simulink model "Simulation_full_Matlab"  (R2024b)
settings: Solver=ode23tb  StartTime=0.0  StopTime=10  MaxStep=1e-5  RelTol=1e-4
InitFcn:
  | Motor_data_IM_R;
undefined symbols (not defined in the file): DiscIntNeverNeededParam, f_n, imr_min, J, j, K_r, K_s, ki, Ki_flux, Ki_w, kp, Kp_flux, Kp_w, L_sigma_r, L_sigma_s, lim, p, P_IN_VA, P_m_n, R_r, R_s, Tau_r, Ts, V_dc, V_ll_n, w_n, wr_n
libraries: slpidlib x2, spsCurrentMeasurementLib x2, spsAsynchronousMachineSIUnitsLib x1, spsDCVoltageSourceLib x1, simulink x1, spsSeriesRLCBranchLib x1, spsUniversalBridgeLib x1, sps_lib x1
settings Model: Creator=dario  LastModifiedBy=dario

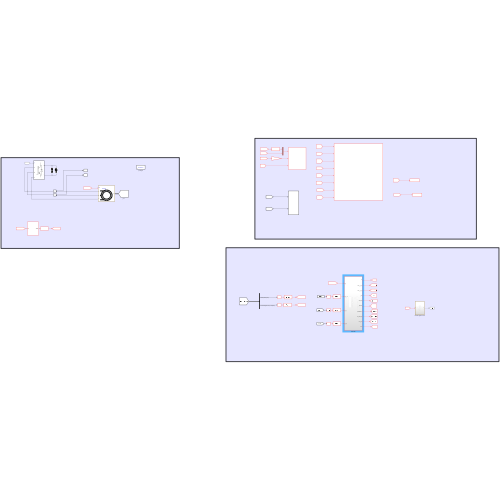
[thumbnail: Simulink's stored preview of the top-level diagram]
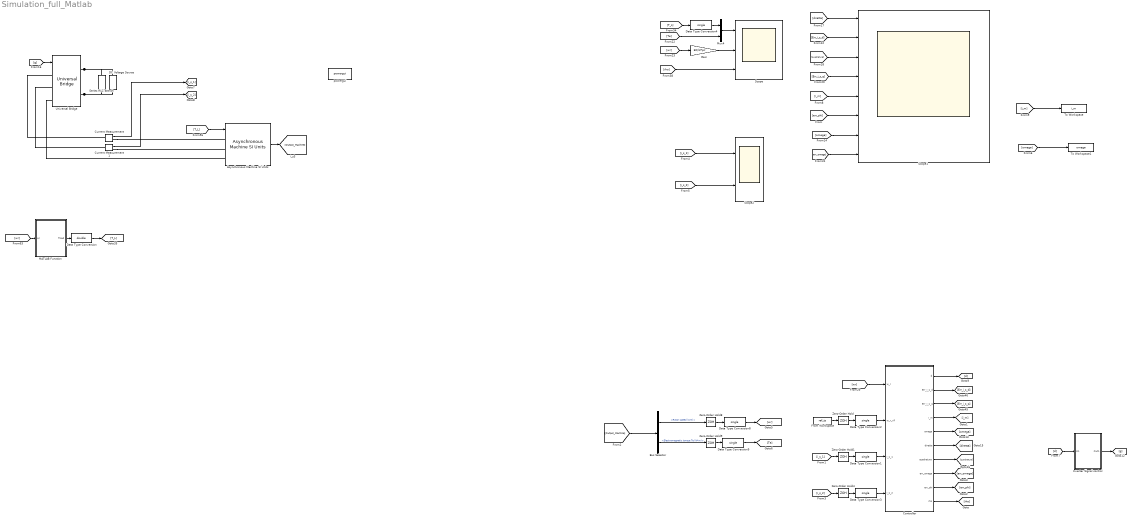
== system Simulation_full_Matlab ==
  Asynchronous Machine SI Units : spsAsynchronousMachineSIUnitsLib/Asynchronous Machine SI Units  RotorType=Squirrel-cage  PresetModel=No  MechanicalLoad=Torque Tm  ShowDetailedParameters=on  ReferenceFrame=Stationary  Units=SI  MeasurementBus=off  NominalParameters=[P_IN_VA V_ll_n f_n]  VoltageRatio=1  Stator=[R_s L_sigma_s]  Rotor=[R_r L_sigma_r]  Cage1=[0.4155 0.002066]  Cage2=[0.4168 0.0003495]  Lm=L_m  Mechanical=[J 0 p]  PolePairs=2  InitialConditions=[1 0 0 0 0 0 -120 -240]  SimulateSaturation=off  Saturation=[14.03593122, 27.81365428, 53.79336849, 72.68890987, 97.98006896, 148.6815601, 215.7428561, 302.9841135, 428.7778367 ; 230, 322, 414, 460, 506, 552, 598, 644, 690]  LoadFlowParameters=1492000  TsPowergui=0  TsBlock=-1  IterativeModel=Trapezoidal non iterative  IterativeDiscreteModel=Trapezoidal non iterative  Pmec=0
  Bus Selector : BusSelector  OutputSignals=Mechanical.Rotor speed (wm),Mechanical.Electromagnetic torque Te (N*m)
  Controller : Subsystem
  Current Measurement : spsCurrentMeasurementLib/Current Measurement  PhasorSimulation=off  OutputType=Complex  PSBequivalent=0
  Current Measurement1 : spsCurrentMeasurementLib/Current Measurement  PhasorSimulation=off  OutputType=Complex  PSBequivalent=0
  DC Voltage Source : spsDCVoltageSourceLib/DC Voltage Source  Amplitude=600  Measurements=None
  Data Type Conversion : DataTypeConversion  OutDataTypeStr=double  SaturateOnIntegerOverflow=off  RndMeth=Floor
  Data Type Conversion{1..4,8..9} (6 alike) : DataTypeConversion  OutDataTypeStr=single  SaturateOnIntegerOverflow=off  RndMeth=Floor
  From Workspace : FromWorkspace  VariableName=ref_ts  OutDataTypeStr=single  Interpolate=off  OutputAfterFinalValue=Holding final value
  Gain : Gain  Gain=60/(2*pi)
  Inverter Signal control : Subsystem
  MATLAB Function : MATLAB Function  TreatAsAtomicUnit=on
  Mux4 : Mux  Inputs=2
  Scope : Scope  NumInputPorts=3
  Scope1 : Scope  NumInputPorts=8
  Scope2 : Scope  NumInputPorts=2
  Series RLC Branch : spsSeriesRLCBranchLib/Series RLC Branch  LConnTagsString=__new0  RConnTagsString=__new0  BranchType=RC  Resistance=0.001  Inductance=1e-3  SetiL0=off  InitialCurrent=0  Capacitance=0.001  Setx0=off  InitialVoltage=0  Measurements=None
  To Workspace : ToWorkspace  VariableName=i_m  SaveFormat=Timeseries  SampleTime=-1
  To Workspace1 : ToWorkspace  VariableName=omega  SaveFormat=Timeseries  SampleTime=-1
  Universal Bridge : spsUniversalBridgeLib/Universal Bridge  Arms=3  SnubberResistance=1e5  SnubberCapacitance=inf  Device=IGBT / Diodes  Ron=1e-3  Lon=0  ForwardVoltages="[  0  0  ]"  ForwardVoltage=0  GTOparameters=[ 10e-6 , 20e-6 ]  IGBTparameters=[ 1e-6 , 2e-6 ]  Measurements=None  Measurements_2=None  converterType=Rectifier
  Zero-Order Hold : ZeroOrderHold  SampleTime=Ts
  Zero-Order Hold{1,4,8..9} (4 alike) : ZeroOrderHold  SampleTime=-1
  powergui : sps_lib/powergui  Priority=1  SimulationMode=Continuous  SampleTime=50e-6  frequency=60  Iterations=50  frequencyindice=50  Pbase=100e6  ErrMax=1e-4  UnitsV=kV  UnitsW=MW  buscounter=0  FunctionMessages=off  echomessages=off  EnableUseOfTLC=off  CurrentSourceSwitches=off  DisableSnubberDevices=off  DisableRonSwitches=off  DisableVfSwitches=off  DisplayEquations=off  AutomaticDiscreteSolvers=off  SolverType=Tustin/Backward Euler (TBE)  Interpol=off  ExternalGateDelay=off  methode=off  Ts=100  x0status=blocks  SPID=on  SwTol=0  HookPort=off  NonlinearTolerance=1e-4  nMaxIteration=100  ContinueOnMaxIteration=off  RestoreLinks=warning  ResistiveCurrentMeasurement=off  Frange=[0:2:500]  Ylog=off  Xlog=on  ShowGrid=off  save=off  variable=ZData  structure=0  ZoomFFT=off  StartTime=0.0  cycles=1  DisplayStyle=1  fundamental=60  FreqAxis=off  MaxFrequency=1000  frequencyindicesteady=1  RmsSteady=1  display=off
  wires:
  Asynchronous Machine SI Units/1 -> [Output_Machine]
  Bus Selector/1 -> Zero-Order Hold8/1  "<Rotor speed (wm)>"
  Bus Selector/2 -> Zero-Order Hold9/1  "<Electromagnetic torque Te (N*m)>"
  [wr] -> Gain/1
  [g] -> Universal Bridge/1
  Current Measurement/1 -> [i_s_1]
  Current Measurement1/1 -> [i_s_2]
  [rho] -> Scope/3
  [Err_i_s_d] -> Scope1/2
  [Err_i_s_q] -> Scope1/4
  [err_phi] -> Scope1/6
  [err_omega] -> Scope1/8
  [T_L] -> Asynchronous Machine SI Units/1
  Mux4/1 -> Scope/1
  [T_L] -> Data Type Conversion4/1
  MATLAB Function/1(Tload) -> Data Type Conversion/1
  [wr] -> MATLAB Function/1(wr)
  Data Type Conversion4/1 -> Mux4/1
  [Output_Machine] -> Bus Selector/1
  Data Type Conversion8/1 -> [wr]
  Data Type Conversion9/1 -> [Te]
  Zero-Order Hold8/1 -> Data Type Conversion8/1
  Zero-Order Hold9/1 -> Data Type Conversion9/1
  [i_m] -> Scope1/5
  [omega] -> Scope1/7
  [diretta] -> Scope1/1
  [quadratura] -> Scope1/3
  [wr] -> Controller/1(w_r)
  From Workspace/1 -> Zero-Order Hold/1
  [i_s_1] -> Zero-Order Hold1/1
  [i_s_2] -> Zero-Order Hold4/1
  Controller/1(d) -> [d]
  [d] -> Inverter Signal control/1(In1)
  Inverter Signal control/1(Out1) -> [g]
  Controller/2(Err_i_s_d) -> [Err_i_s_d]
  Controller/3(Err_i_s_q) -> [Err_i_s_q]
  Controller/4(i_m) -> [i_m]
  Controller/5(omega) -> [omega]
  Controller/6(diretta) -> [diretta]
  Controller/7(quadratura) -> [quadratura]
  Controller/9(err_phi) -> [err_phi]
  Controller/10(rho) -> [rho]
  Controller/8(err_omega) -> [err_omega]
  [Te] -> Mux4/2
  Gain/1 -> Scope/2
  [i_s_1] -> Scope2/1
  [i_s_2] -> Scope2/2
  Zero-Order Hold1/1 -> Data Type Conversion1/1
  Data Type Conversion1/1 -> Controller/3(i_s_1)
  Data Type Conversion3/1 -> Controller/4(i_s_2)
  Zero-Order Hold4/1 -> Data Type Conversion3/1
  Zero-Order Hold/1 -> Data Type Conversion2/1
  Data Type Conversion2/1 -> Controller/2(w_r_rif)
  Data Type Conversion/1 -> [T_L]
  [i_m] -> To Workspace/1
  [omega] -> To Workspace1/1
  connections:
  Current Measurement/LConn1 -- Universal Bridge/LConn1
  Universal Bridge/LConn2 -- Current Measurement1/LConn1
  Universal Bridge/RConn1 -- DC Voltage Source/RConn1 -- Series RLC Branch/LConn1
  Universal Bridge/RConn2 -- DC Voltage Source/LConn1 -- Series RLC Branch/RConn1
  Current Measurement/RConn1 -- Asynchronous Machine SI Units/LConn1
  Current Measurement1/RConn1 -- Asynchronous Machine SI Units/LConn2
  Universal Bridge/LConn3 -- Asynchronous Machine SI Units/LConn3

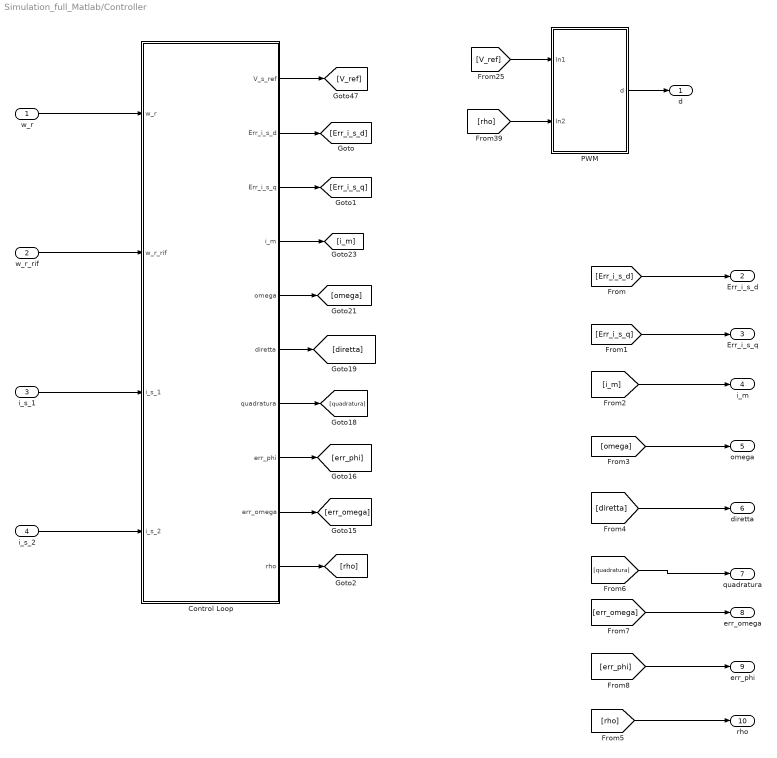
== system Simulation_full_Matlab/Controller ==
  w_r : Inport
  w_r_rif : Inport  Port=2
  i_s_1 : Inport  Port=3
  i_s_2 : Inport  Port=4
  Control Loop : Subsystem
  PWM : Subsystem
  d : Outport
  Err_i_s_d : Outport  Port=2
  Err_i_s_q : Outport  Port=3
  i_m : Outport  Port=4
  omega : Outport  Port=5
  diretta : Outport  Port=6
  quadratura : Outport  Port=7
  err_omega : Outport  Port=8
  err_phi : Outport  Port=9
  rho : Outport  Port=10
  wires:
  w_r/1 -> Control Loop/1(w_r)
  Control Loop/1(V_s_ref) -> [V_ref]
  w_r_rif/1 -> Control Loop/2(w_r_rif)
  i_s_1/1 -> Control Loop/3(i_s_1)
  i_s_2/1 -> Control Loop/4(i_s_2)
  [V_ref] -> PWM/1(In1)
  PWM/1(d) -> d/1
  [rho] -> PWM/2(In2)
  [Err_i_s_q] -> Err_i_s_q/1
  [Err_i_s_d] -> Err_i_s_d/1
  [quadratura] -> quadratura/1
  [i_m] -> i_m/1
  [diretta] -> diretta/1
  [omega] -> omega/1
  Control Loop/2(Err_i_s_d) -> [Err_i_s_d]
  Control Loop/3(Err_i_s_q) -> [Err_i_s_q]
  Control Loop/4(i_m) -> [i_m]
  Control Loop/5(omega) -> [omega]
  Control Loop/6(diretta) -> [diretta]
  Control Loop/7(quadratura) -> [quadratura]
  Control Loop/8(err_phi) -> [err_phi]
  Control Loop/9(err_omega) -> [err_omega]
  Control Loop/10(rho) -> [rho]
  [rho] -> rho/1
  [err_omega] -> err_omega/1
  [err_phi] -> err_phi/1

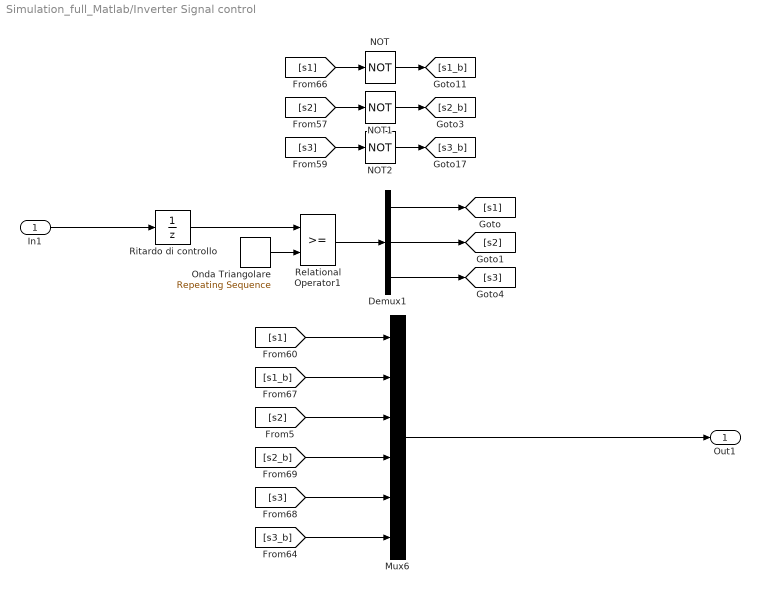
== system Simulation_full_Matlab/Inverter Signal control ==
  In1 : Inport
  Demux1 : Demux  Outputs=3
  Mux6 : Mux  Inputs=6
  NOT : Logic  Operator=NOT  IconShape=distinctive  AllPortsSameDT=off  OutDataTypeStr=boolean
  NOT1 : Logic  Operator=NOT  IconShape=distinctive  AllPortsSameDT=off  OutDataTypeStr=boolean
  NOT2 : Logic  Operator=NOT  IconShape=distinctive  AllPortsSameDT=off  OutDataTypeStr=boolean
  Onda Triangolare : simulink/Sources/Repeating Sequence  rep_seq_t=[0 Ts/2 Ts]  rep_seq_y=[0 1 0]
  Relational Operator1 : RelationalOperator  OutDataTypeStr=boolean  RndMeth=Simplest  InputSameDT=off
  Ritardo di controllo : UnitDelay  SampleTime=Ts  HasFrameUpgradeWarning=on
  Out1 : Outport
  wires:
  Onda Triangolare/1 -> Relational Operator1/2
  Mux6/1 -> Out1/1
  NOT/1 -> [s1_b]
  NOT1/1 -> [s2_b]
  [s2_b] -> Mux6/4
  In1/1 -> Ritardo di controllo/1
  [s3] -> Mux6/5
  Ritardo di controllo/1 -> Relational Operator1/1
  [s2] -> Mux6/3
  Relational Operator1/1 -> Demux1/1
  [s1_b] -> Mux6/2
  [s2] -> NOT1/1
  Demux1/2 -> [s2]
  [s3_b] -> Mux6/6
  Demux1/3 -> [s3]
  [s1] -> NOT/1
  NOT2/1 -> [s3_b]
  [s1] -> Mux6/1
  [s3] -> NOT2/1
  Demux1/1 -> [s1]

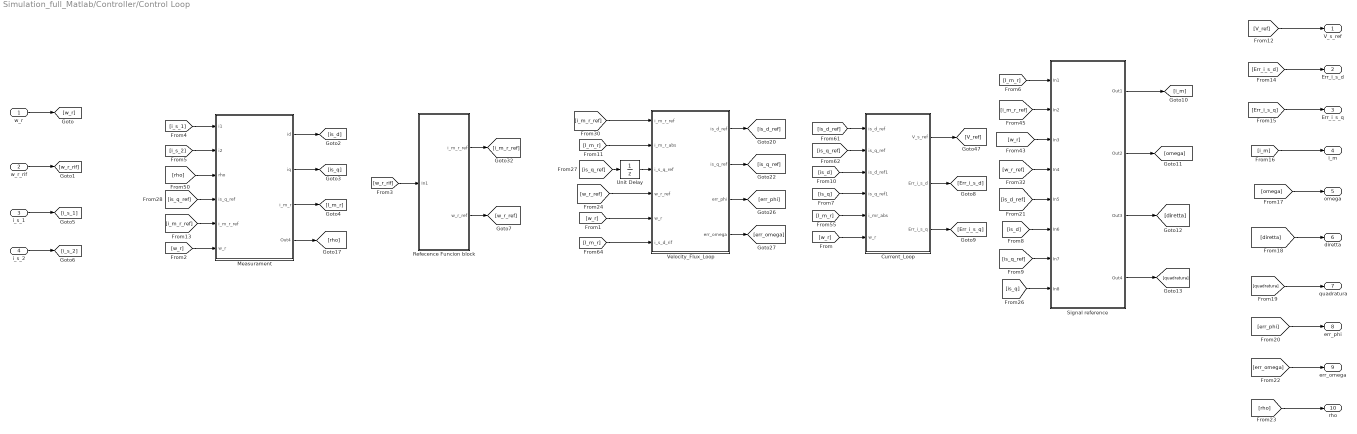
== system Simulation_full_Matlab/Controller/Control Loop ==
  w_r : Inport
  w_r_rif : Inport  Port=2
  i_s_1 : Inport  Port=3
  i_s_2 : Inport  Port=4
  Current_Loop : Subsystem
  Measurament : Subsystem
  Refecence Funcion block : Subsystem
  Signal reference : Subsystem
  Unit Delay : UnitDelay  SampleTime=-1  HasFrameUpgradeWarning=on
  Velocity_Flux_Loop : Subsystem
  V_s_ref : Outport
  Err_i_s_d : Outport  Port=2
  Err_i_s_q : Outport  Port=3
  i_m : Outport  Port=4
  omega : Outport  Port=5
  diretta : Outport  Port=6
  quadratura : Outport  Port=7
  err_phi : Outport  Port=8
  err_omega : Outport  Port=9
  rho : Outport  Port=10
  wires:
  Velocity_Flux_Loop/3(err_phi) -> [err_phi]
  [is_d_ref] -> Current_Loop/1(is_d_ref)
  [is_q] -> Current_Loop/4(is_q_ref1)
  [is_q_ref] -> Unit Delay/1
  [w_r_ref] -> Velocity_Flux_Loop/4(w_r_ref)
  [i_m_r_ref] -> Velocity_Flux_Loop/1(i_m_r_ref)
  [I_m_r] -> Velocity_Flux_Loop/2(i_m_r_abs)
  [is_d] -> Current_Loop/3(is_d_ref1)
  Velocity_Flux_Loop/4(err_omega) -> [err_omega]
  Velocity_Flux_Loop/2(is_q_ref) -> [is_q_ref]
  Velocity_Flux_Loop/1(is_d_ref) -> [is_d_ref]
  [I_m_r] -> Current_Loop/5(i_mr_abs)
  [is_q_ref] -> Current_Loop/2(is_q_ref)
  Unit Delay/1 -> Velocity_Flux_Loop/3(i_s_q_ref)
  [I_m_r] -> Velocity_Flux_Loop/6(i_s_d_rif)
  w_r/1 -> [w_r]
  [w_r] -> Velocity_Flux_Loop/5(w_r)
  [w_r] -> Current_Loop/6(w_r)
  w_r_rif/1 -> [w_r_rif]
  i_s_1/1 -> [i_s_1]
  i_s_2/1 -> [i_s_2]
  [w_r_rif] -> Refecence Funcion block/1(In1)
  Refecence Funcion block/1(i_m_r_ref) -> [i_m_r_ref]
  [i_s_1] -> Measurament/1(i1)
  [i_s_2] -> Measurament/2(i2)
  [rho] -> Measurament/3(rho)
  [is_q_ref] -> Measurament/4(is_q_ref)
  [i_m_r_ref] -> Measurament/5(i_m_r_ref)
  [w_r] -> Measurament/6(w_r)
  Measurament/1(id) -> [is_d]
  Measurament/2(iq) -> [is_q]
  Measurament/3(i_m_r) -> [I_m_r]
  Measurament/4(Out4) -> [rho]
  Refecence Funcion block/2(w_r_ref) -> [w_r_ref]
  Current_Loop/1(V_s_ref) -> [V_ref]
  Current_Loop/2(Err_i_s_d) -> [Err_i_s_d]
  Current_Loop/3(Err_i_s_q) -> [Err_i_s_q]
  [V_ref] -> V_s_ref/1
  [Err_i_s_d] -> Err_i_s_d/1
  [Err_i_s_q] -> Err_i_s_q/1
  [I_m_r] -> Signal reference/1(In1)
  [i_m_r_ref] -> Signal reference/2(In2)
  [w_r] -> Signal reference/3(In3)
  [w_r_ref] -> Signal reference/4(In4)
  [is_d_ref] -> Signal reference/5(In5)
  [is_d] -> Signal reference/6(In6)
  [is_q_ref] -> Signal reference/7(In7)
  [is_q] -> Signal reference/8(In8)
  Signal reference/1(Out1) -> [i_m]
  Signal reference/2(Out2) -> [omega]
  Signal reference/3(Out3) -> [diretta]
  Signal reference/4(Out4) -> [quadratura]
  [omega] -> omega/1
  [i_m] -> i_m/1
  [diretta] -> diretta/1
  [quadratura] -> quadratura/1
  [err_phi] -> err_phi/1
  [err_omega] -> err_omega/1
  [rho] -> rho/1

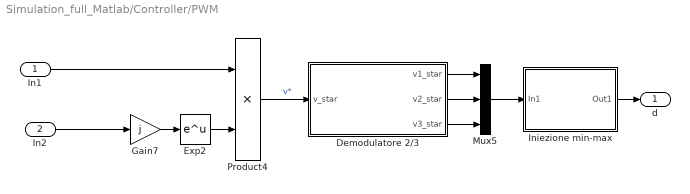
== system Simulation_full_Matlab/Controller/PWM ==
  In1 : Inport
  In2 : Inport  Port=2
  Demodulatore 2/3 : MATLAB Function  TreatAsAtomicUnit=on
  Exp2 : Math  SignedPower=on
  Gain7 : Gain  Gain=j
  Iniezione min-max : Subsystem
  Mux5 : Mux  Inputs=3
  Product4 : Product
  d : Outport
  wires:
  Mux5/1 -> Iniezione min-max/1(In1)
  Demodulatore 2/3/2(v2_star) -> Mux5/2
  Demodulatore 2/3/3(v3_star) -> Mux5/3
  Demodulatore 2/3/1(v1_star) -> Mux5/1
  Iniezione min-max/1(Out1) -> d/1
  Exp2/1 -> Product4/2
  Gain7/1 -> Exp2/1
  In2/1 -> Gain7/1
  Product4/1 -> Demodulatore 2/3/1(v_star)  "v*"
  In1/1 -> Product4/1

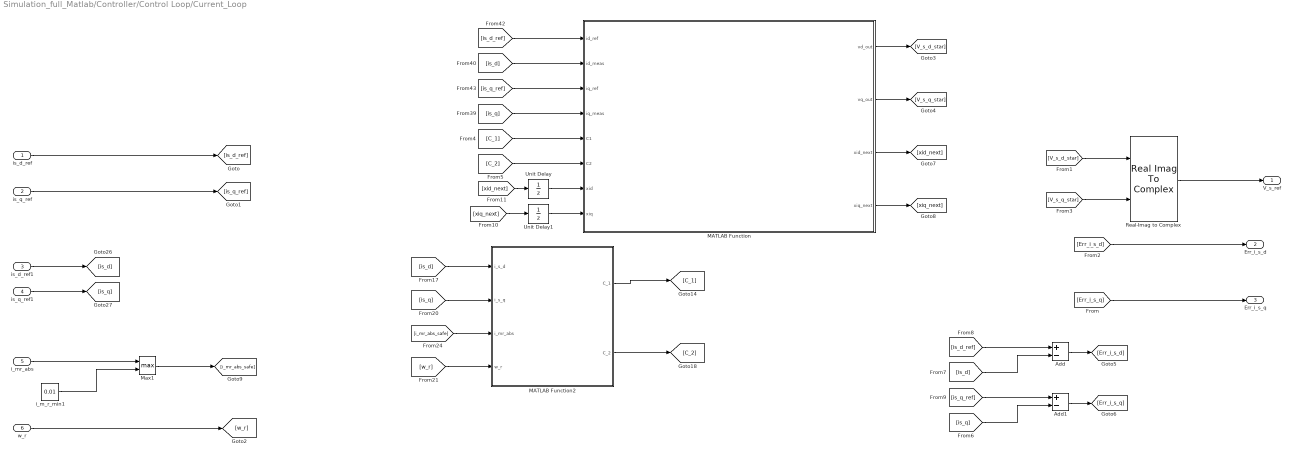
== system Simulation_full_Matlab/Controller/Control Loop/Current_Loop ==
  is_d_ref : Inport
  is_q_ref : Inport  Port=2
  is_d_ref1 : Inport  Port=3
  is_q_ref1 : Inport  Port=4
  i_mr_abs : Inport  Port=5
  w_r : Inport  Port=6
  Add : Sum  Inputs=+-
  Add1 : Sum  Inputs=+-
  MATLAB Function : MATLAB Function  TreatAsAtomicUnit=on  mask{Kp_d=kp, Ki_d=ki, Kp_q=kp, Ki_q=ki}
  MATLAB Function2 : MATLAB Function  TreatAsAtomicUnit=on
  Max1 : MinMax  Function=max  Inputs=2
  Real-Imag to Complex : RealImagToComplex
  Unit Delay : UnitDelay  SampleTime=-1  HasFrameUpgradeWarning=on
  Unit Delay1 : UnitDelay  SampleTime=-1  HasFrameUpgradeWarning=on
  i_m_r_min1 : Constant  Value=0.01  OutDataTypeStr=single
  V_s_ref : Outport
  Err_i_s_d : Outport  Port=2
  Err_i_s_q : Outport  Port=3
  wires:
  is_q_ref1/1 -> [is_q]
  [w_r] -> MATLAB Function2/4(w_r)
  [is_q] -> MATLAB Function2/2(i_s_q)
  [is_d] -> MATLAB Function2/1(i_s_d)
  [i_mr_abs_safe] -> MATLAB Function2/3(i_mr_abs)
  Max1/1 -> [i_mr_abs_safe]
  i_m_r_min1/1 -> Max1/2
  MATLAB Function2/2(C_2) -> [C_2]
  is_d_ref1/1 -> [is_d]
  MATLAB Function2/1(C_1) -> [C_1]
  i_mr_abs/1 -> Max1/1
  is_d_ref/1 -> [is_d_ref]
  is_q_ref/1 -> [is_q_ref]
  w_r/1 -> [w_r]
  [Err_i_s_d] -> Err_i_s_d/1
  [Err_i_s_q] -> Err_i_s_q/1
  Real-Imag to Complex/1 -> V_s_ref/1
  [V_s_d_star] -> Real-Imag to Complex/1
  [V_s_q_star] -> Real-Imag to Complex/2
  [is_d_ref] -> MATLAB Function/1(id_ref)
  [is_d] -> MATLAB Function/2(id_meas)
  [is_q_ref] -> MATLAB Function/3(iq_ref)
  [is_q] -> MATLAB Function/4(iq_meas)
  [C_1] -> MATLAB Function/5(C1)
  [C_2] -> MATLAB Function/6(C2)
  MATLAB Function/1(vd_out) -> [V_s_d_star]
  MATLAB Function/2(vq_out) -> [V_s_q_star]
  [is_d] -> Add/2
  [is_d_ref] -> Add/1
  Add/1 -> [Err_i_s_d]
  [is_q_ref] -> Add1/1
  Add1/1 -> [Err_i_s_q]
  [is_q] -> Add1/2
  MATLAB Function/3(xid_next) -> [xid_next]
  MATLAB Function/4(xiq_next) -> [xiq_next]
  [xid_next] -> Unit Delay/1
  Unit Delay/1 -> MATLAB Function/7(xid)
  [xiq_next] -> Unit Delay1/1
  Unit Delay1/1 -> MATLAB Function/8(xiq)

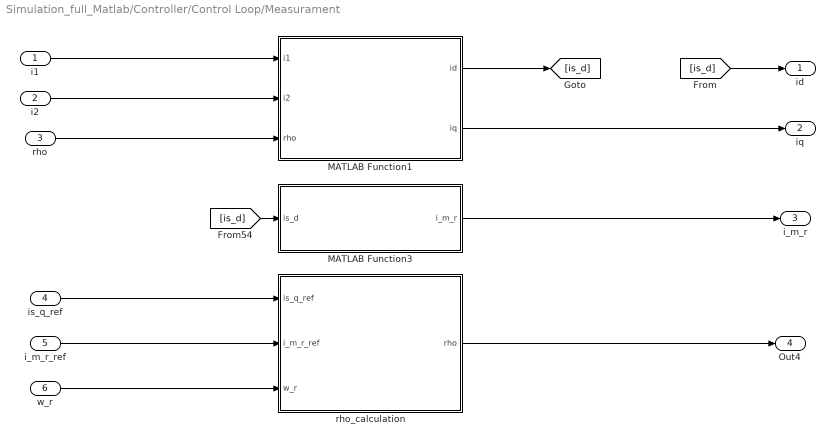
== system Simulation_full_Matlab/Controller/Control Loop/Measurament ==
  i1 : Inport
  i2 : Inport  Port=2
  rho : Inport  Port=3
  is_q_ref : Inport  Port=4
  i_m_r_ref : Inport  Port=5
  w_r : Inport  Port=6
  MATLAB Function1 : MATLAB Function  TreatAsAtomicUnit=on
  MATLAB Function3 : MATLAB Function  TreatAsAtomicUnit=on
  rho_calculation : Subsystem
  id : Outport
  iq : Outport  Port=2
  i_m_r : Outport  Port=3
  Out4 : Outport  Port=4
  wires:
  MATLAB Function3/1(i_m_r) -> i_m_r/1
  i2/1 -> MATLAB Function1/2(i2)
  [is_d] -> MATLAB Function3/1(is_d)
  i1/1 -> MATLAB Function1/1(i1)
  w_r/1 -> rho_calculation/3(w_r)
  MATLAB Function1/2(iq) -> iq/1
  MATLAB Function1/1(id) -> [is_d]
  i_m_r_ref/1 -> rho_calculation/2(i_m_r_ref)
  rho/1 -> MATLAB Function1/3(rho)
  rho_calculation/1(rho) -> Out4/1
  is_q_ref/1 -> rho_calculation/1(is_q_ref)
  [is_d] -> id/1

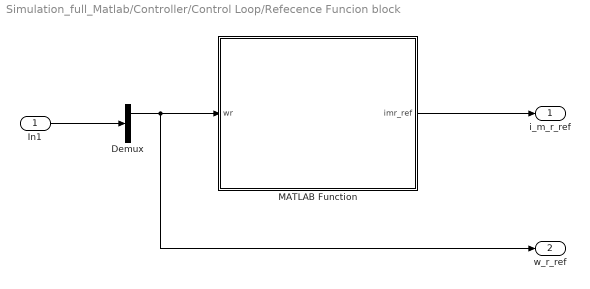
== system Simulation_full_Matlab/Controller/Control Loop/Refecence Funcion block ==
  In1 : Inport
  Demux : Demux  Outputs=2
  MATLAB Function : MATLAB Function  TreatAsAtomicUnit=on
  i_m_r_ref : Outport
  w_r_ref : Outport  Port=2
  wires:
  MATLAB Function/1(imr_ref) -> i_m_r_ref/1
  Demux/1 -> w_r_ref/1, MATLAB Function/1(wr)
  In1/1 -> Demux/1

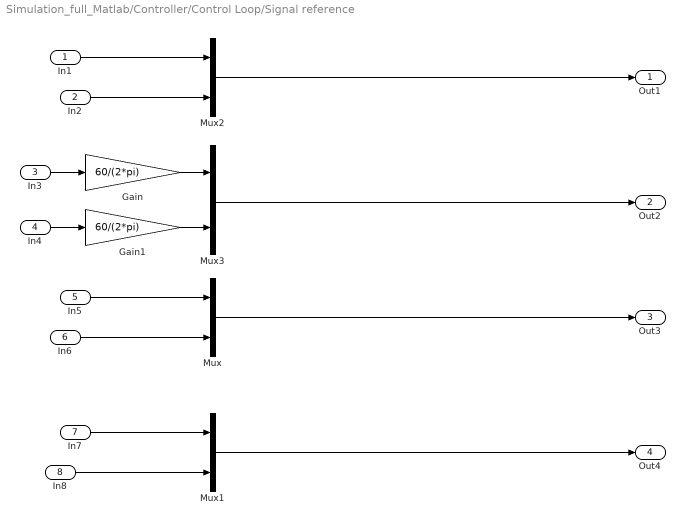
== system Simulation_full_Matlab/Controller/Control Loop/Signal reference ==
  In1 : Inport
  In2 : Inport  Port=2
  In3 : Inport  Port=3
  In4 : Inport  Port=4
  In5 : Inport  Port=5
  In6 : Inport  Port=6
  In7 : Inport  Port=7
  In8 : Inport  Port=8
  Gain : Gain  Gain=60/(2*pi)
  Gain1 : Gain  Gain=60/(2*pi)
  Mux{,1..3} (4 alike) : Mux  Inputs=2
  Out1 : Outport
  Out2 : Outport  Port=2
  Out3 : Outport  Port=3
  Out4 : Outport  Port=4
  wires:
  In8/1 -> Mux1/2
  In1/1 -> Mux2/1
  Mux2/1 -> Out1/1
  In6/1 -> Mux/2
  In5/1 -> Mux/1
  In2/1 -> Mux2/2
  Mux/1 -> Out3/1
  Mux1/1 -> Out4/1
  In4/1 -> Gain1/1
  In3/1 -> Gain/1
  In7/1 -> Mux1/1
  Mux3/1 -> Out2/1
  Gain/1 -> Mux3/1
  Gain1/1 -> Mux3/2

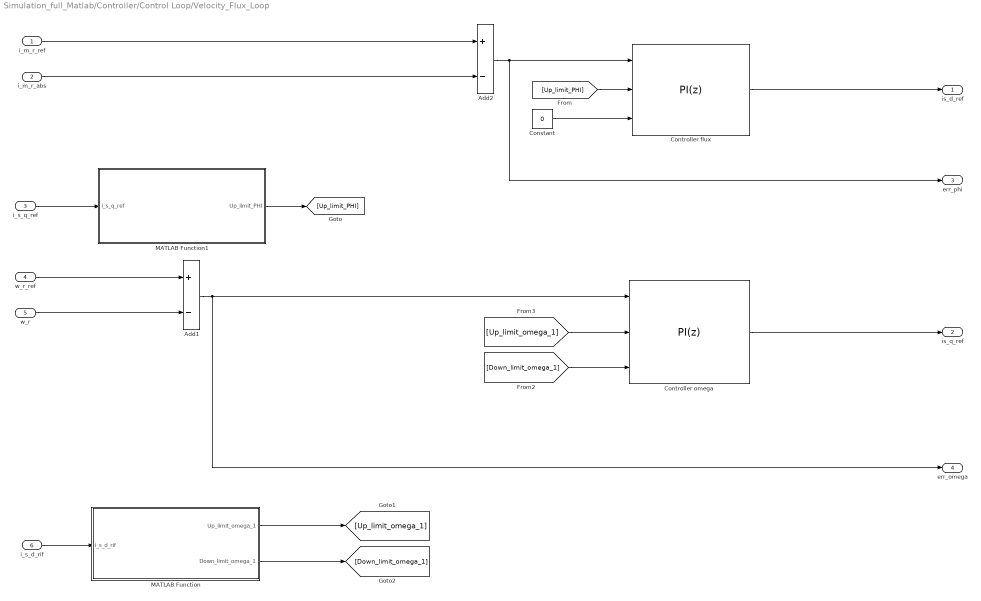
== system Simulation_full_Matlab/Controller/Control Loop/Velocity_Flux_Loop ==
  i_m_r_ref : Inport
  i_m_r_abs : Inport  Port=2
  i_s_q_ref : Inport  Port=3
  w_r_ref : Inport  Port=4
  w_r : Inport  Port=5
  i_s_d_rif : Inport  Port=6
  Add1 : Sum  Inputs=+-
  Add2 : Sum  Inputs=+-
  Constant : Constant  Value=0  OutDataTypeStr=single
  Controller flux : slpidlib/PID Controller  Controller=PI  Form=Parallel  TimeDomain=Discrete-time  UseExternalTs=off  SampleTime=-1  IntegratorMethod=Trapezoidal  FilterMethod=Forward Euler  ControllerParametersSource=internal  P=10*Kp_flux  I=4*Ki_flux  UseKiTs=off  D=0  UseExternalDerivativeSource=off  N=100  UseFilter=on  TunerSelectOption=Transfer Function Based (PID Tuner App)  InitialConditionSource=internal  InitialConditionForIntegrator=0  InitialConditionForFilter=0  DifferentiatorICPrevScaledInput=0  ExternalReset=none  TrackingMode=off  Kt=1  LimitOutput=on  SatLimitsSource=external  UpperSaturationLimit=inf  LowerSaturationLimit=-inf  LinearizeAsGain=on  AntiWindupMode=clamping  Kb=1  LimitIntegrator=off  UpperIntegratorSaturationLimit=Up_limit_PHI  LowerIntegratorSaturationLimit=0  POutMin=[]  POutMax=[]  IOutMin=[]  IOutMax=[]  DOutMin=[]  DOutMax=[]  NOutMin=[]  NOutMax=[]  SumOutMin=[]  SumOutMax=[]  SaturationOutMin=[]  SaturationOutMax=[]  PParamMin=[]  PParamMax=[]  IParamMin=[]  IParamMax=[]  DParamMin=[]  DParamMax=[]  NParamMin=[]  NParamMax=[]  KbParamMin=[]  KbParamMax=[]  KtParamMin=[]  KtParamMax=[]  KbOutMin=[]  KbOutMax=[]  KtOutMin=[]  KtOutMax=[]  IntegratorOutMin=[]  IntegratorOutMax=[]  FilterOutMin=[]  FilterOutMax=[]  SumI1OutMin=[]  SumI1OutMax=[]  SumI2OutMin=[]  SumI2OutMax=[]  SumI3OutMin=[]  SumI3OutMax=[]  SumI4OutMin=[]  SumI4OutMax=[]  SumDOutMin=[]  SumDOutMax=[]  DifferentiatorOutMin=[]  DifferentiatorOutMax=[]  FilterDiffOutCoefMin=[]  FilterDiffOutCoefMax=[]  ReciprocalOutMin=[]  ReciprocalOutMax=[]  SumDenOutMin=[]  SumDenOutMax=[]  SumNumOutMin=[]  SumNumOutMax=[]  DivideOutMin=[]  DivideOutMax=[]  UdiffTsProdOutMin=[]  UdiffTsProdOutMax=[]  NTsProdOutMin=[]  NTsProdOutMax=[]  UintegralTsProdOutMin=[]  UintegralTsProdOutMax=[]  UngainTsProdOutMin=[]  UngainTsProdOutMax=[]  ClampingZeroOutDataTypeStr=Inherit: Inherit via back propagation  ClampingZeroOutMin=[]  ClampingZeroOutMax=[]  FilterDenConstantOutDataTypeStr=Inherit: Inherit via back propagation  FilterDenConstantOutMin=[]  FilterDenConstantOutMax=[]  PCopyOutDataTypeStr=Inherit: Inherit via back propagation  PCopyOutMin=[]  PCopyOutMax=[]  NCopyOutDataTypeStr=Inherit: Inherit via back propagation  NCopyOutMin=[]  NCopyOutMax=[]  IntegratorContinuousStateAttributes=''  IntegratorStateMustResolveToSignalObject=off  IntegratorRTWStateStorageClass=Auto  FilterContinuousStateAttributes=''  FilterStateMustResolveToSignalObject=off  FilterRTWStateStorageClass=Auto  ParallelPVariant=InternalParameters  IdealPVariant=Disabled  IVariant=InternalParameters  DVariant=Disabled  IntegratorVariant=Discrete  SatVariant=External  AWVariant=DiscClampingParallel  PCopyVariant=Disabled  TRVariant=Disabled  FdbkBlocksVariant=Feedback  IdealPFdbkVariant=Passthrough  SatFdbkVariant=Passthrough  DerivativeFilterVariant=Disabled  NVariant=Disabled  NCopyVariant=Disabled_SignalSpec  FilterICVariant=Disabled  IntegratorICVariant=InternalICs  ExternalResetVariant=Disabled  TRSumVariant=Passthrough  SumFdbkVariant=Enabled  SumVariant=Sum_PI  TsampFilterVariant=InternalTs  TsampNgainVariant=Passthrough  TsampIntegralVariant=Disabled_SignalSpec  ExternalSaturationOutDataTypeStr=Inherit: Same as second input  DerivativeSourceVariant=Disabled  PreIntVariant=InternalPreInt
  Controller omega : slpidlib/PID Controller  Controller=PI  Form=Parallel  TimeDomain=Discrete-time  UseExternalTs=off  SampleTime=-1  IntegratorMethod=Trapezoidal  FilterMethod=Forward Euler  ControllerParametersSource=internal  P=3*Kp_w  I=1*Ki_w  UseKiTs=off  D=0  UseExternalDerivativeSource=off  N=100  UseFilter=on  TunerSelectOption=Transfer Function Based (PID Tuner App)  InitialConditionSource=internal  InitialConditionForIntegrator=0  InitialConditionForFilter=0  DifferentiatorICPrevScaledInput=0  ExternalReset=none  TrackingMode=off  Kt=1  LimitOutput=on  SatLimitsSource=external  UpperSaturationLimit=inf  LowerSaturationLimit=-inf  LinearizeAsGain=on  AntiWindupMode=clamping  Kb=1  LimitIntegrator=off  UpperIntegratorSaturationLimit=Up_limit_PHI  LowerIntegratorSaturationLimit=0  POutMin=[]  POutMax=[]  IOutMin=[]  IOutMax=[]  DOutMin=[]  DOutMax=[]  NOutMin=[]  NOutMax=[]  SumOutMin=[]  SumOutMax=[]  SaturationOutMin=[]  SaturationOutMax=[]  PParamMin=[]  PParamMax=[]  IParamMin=[]  IParamMax=[]  DParamMin=[]  DParamMax=[]  NParamMin=[]  NParamMax=[]  KbParamMin=[]  KbParamMax=[]  KtParamMin=[]  KtParamMax=[]  KbOutMin=[]  KbOutMax=[]  KtOutMin=[]  KtOutMax=[]  IntegratorOutMin=[]  IntegratorOutMax=[]  FilterOutMin=[]  FilterOutMax=[]  SumI1OutMin=[]  SumI1OutMax=[]  SumI2OutMin=[]  SumI2OutMax=[]  SumI3OutMin=[]  SumI3OutMax=[]  SumI4OutMin=[]  SumI4OutMax=[]  SumDOutMin=[]  SumDOutMax=[]  DifferentiatorOutMin=[]  DifferentiatorOutMax=[]  FilterDiffOutCoefMin=[]  FilterDiffOutCoefMax=[]  ReciprocalOutMin=[]  ReciprocalOutMax=[]  SumDenOutMin=[]  SumDenOutMax=[]  SumNumOutMin=[]  SumNumOutMax=[]  DivideOutMin=[]  DivideOutMax=[]  UdiffTsProdOutMin=[]  UdiffTsProdOutMax=[]  NTsProdOutMin=[]  NTsProdOutMax=[]  UintegralTsProdOutMin=[]  UintegralTsProdOutMax=[]  UngainTsProdOutMin=[]  UngainTsProdOutMax=[]  ClampingZeroOutDataTypeStr=Inherit: Inherit via back propagation  ClampingZeroOutMin=[]  ClampingZeroOutMax=[]  FilterDenConstantOutDataTypeStr=Inherit: Inherit via back propagation  FilterDenConstantOutMin=[]  FilterDenConstantOutMax=[]  PCopyOutDataTypeStr=Inherit: Inherit via back propagation  PCopyOutMin=[]  PCopyOutMax=[]  NCopyOutDataTypeStr=Inherit: Inherit via back propagation  NCopyOutMin=[]  NCopyOutMax=[]  IntegratorContinuousStateAttributes=''  IntegratorStateMustResolveToSignalObject=off  IntegratorRTWStateStorageClass=Auto  FilterContinuousStateAttributes=''  FilterStateMustResolveToSignalObject=off  FilterRTWStateStorageClass=Auto  ParallelPVariant=InternalParameters  IdealPVariant=Disabled  IVariant=InternalParameters  DVariant=Disabled  IntegratorVariant=Discrete  SatVariant=External  AWVariant=DiscClampingParallel  PCopyVariant=Disabled  TRVariant=Disabled  FdbkBlocksVariant=Feedback  IdealPFdbkVariant=Passthrough  SatFdbkVariant=Passthrough  DerivativeFilterVariant=Disabled  NVariant=Disabled  NCopyVariant=Disabled_SignalSpec  FilterICVariant=Disabled  IntegratorICVariant=InternalICs  ExternalResetVariant=Disabled  TRSumVariant=Passthrough  SumFdbkVariant=Enabled  SumVariant=Sum_PI  TsampFilterVariant=InternalTs  TsampNgainVariant=Passthrough  TsampIntegralVariant=Disabled_SignalSpec  ExternalSaturationOutDataTypeStr=Inherit: Same as second input  DerivativeSourceVariant=Disabled  PreIntVariant=InternalPreInt
  MATLAB Function : MATLAB Function  TreatAsAtomicUnit=on
  MATLAB Function1 : MATLAB Function  TreatAsAtomicUnit=on
  is_d_ref : Outport
  is_q_ref : Outport  Port=2
  err_phi : Outport  Port=3
  err_omega : Outport  Port=4
  wires:
  i_m_r_ref/1 -> Add2/1
  w_r/1 -> Add1/2
  i_m_r_abs/1 -> Add2/2
  Add2/1 -> err_phi/1, Controller flux/1
  Add1/1 -> Controller omega/1, err_omega/1
  w_r_ref/1 -> Add1/1
  Controller omega/1 -> is_q_ref/1
  Controller flux/1 -> is_d_ref/1
  Constant/1 -> Controller flux/3
  [Up_limit_PHI] -> Controller flux/2
  [Up_limit_omega_1] -> Controller omega/2
  [Down_limit_omega_1] -> Controller omega/3
  i_s_d_rif/1 -> MATLAB Function/1(i_s_d_rif)
  MATLAB Function/1(Up_limit_omega_1) -> [Up_limit_omega_1]
  MATLAB Function/2(Down_limit_omega_1) -> [Down_limit_omega_1]
  i_s_q_ref/1 -> MATLAB Function1/1(i_s_q_ref)
  MATLAB Function1/1(Up_limit_PHI) -> [Up_limit_PHI]

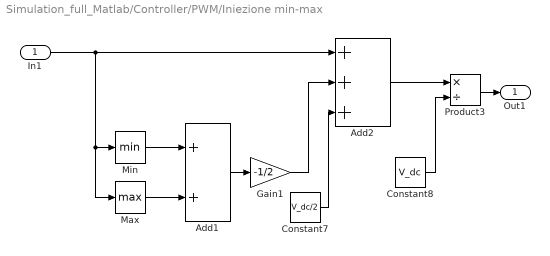
== system Simulation_full_Matlab/Controller/PWM/Iniezione min-max ==
  In1 : Inport
  Add1 : Sum
  Add2 : Sum  Inputs=+++
  Constant7 : Constant  Value=V_dc/2
  Constant8 : Constant  Value=V_dc
  Gain1 : Gain  Gain=-1/2
  Max : MinMax  Function=max
  Min : MinMax
  Product3 : Product  Inputs=*/
  Out1 : Outport
  wires:
  Max/1 -> Add1/2
  Constant7/1 -> Add2/3
  Constant8/1 -> Product3/2
  Min/1 -> Add1/1
  In1/1 -> Max/1, Min/1, Add2/1
  Add1/1 -> Gain1/1
  Gain1/1 -> Add2/2
  Add2/1 -> Product3/1
  Product3/1 -> Out1/1

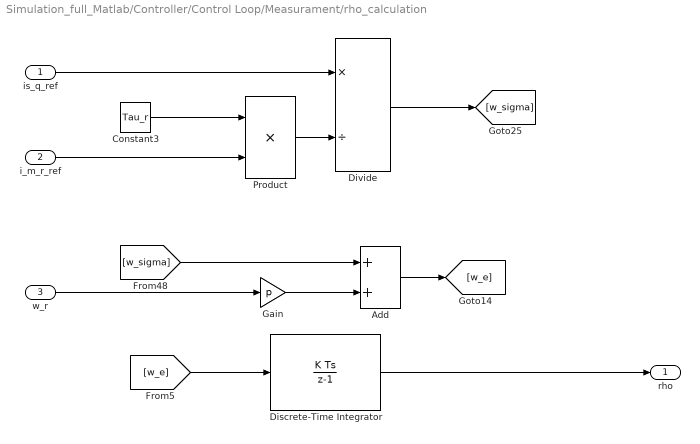
== system Simulation_full_Matlab/Controller/Control Loop/Measurament/rho_calculation ==
  is_q_ref : Inport
  i_m_r_ref : Inport  Port=2
  w_r : Inport  Port=3
  Add : Sum
  Constant3 : Constant  Value=Tau_r
  Discrete-Time Integrator : DiscreteIntegrator  SampleTime=-1  OutDataTypeStr=single  ICPrevOutput=DiscIntNeverNeededParam  ICPrevScaledInput=DiscIntNeverNeededParam
  Divide : Product  Inputs=*/
  Gain : Gain  Gain=p
  Product : Product
  rho : Outport
  wires:
  Gain/1 -> Add/2
  Product/1 -> Divide/2
  Divide/1 -> [w_sigma]
  Constant3/1 -> Product/1
  [w_sigma] -> Add/1
  Add/1 -> [w_e]
  i_m_r_ref/1 -> Product/2
  [w_e] -> Discrete-Time Integrator/1
  w_r/1 -> Gain/1
  is_q_ref/1 -> Divide/1
  Discrete-Time Integrator/1 -> rho/1

== matlab function Simulation_full_Matlab/Controller/PWM/Demodulatore 2//3 ==
  settings: updateMethod=DISCRETE
  data: v_star input; v1_star output; v2_star output; v3_star output
function [v1_star, v2_star, v3_star] = demodulation(v_star)
v1_star=real(v_star);
v2_star=-1/2*real(v_star)+sqrt(3)/2*imag(v_star);
v3_star=-1/2*real(v_star)-sqrt(3)/2*imag(v_star);

== matlab function Simulation_full_Matlab/MATLAB Function ==
  data: wr input single; Tload output single; w_n parameter single; P_m_n parameter single
function Tload = load_torque(wr, w_n, P_m_n)
% Tload: coppia resistente [N*m]
% wr: velocità meccanica [rad/s]
% w_n: velocità nominale [rad/s]
% P_m_n: potenza nominale [W]
%
% Specifica: |Tload| ∝ |wr|^3 e P(2*w_n)=P_m_n

% Costante K tale che P(2*w_n)=P_m_n
K = P_m_n / (16 * w_n^4);

% Coppia resistente: oppone sempre il moto
Tload = K * wr .* abs(wr).^2;
end

== matlab function Simulation_full_Matlab/Controller/Control Loop/Current_Loop/MATLAB Function ==
  data: id_ref input single; vd_out output single; id_meas input single; iq_ref input single; iq_meas input single; C1 input single; C2 input single; xid input single; xiq input single; vq_out output single; xid_next output single; xiq_next output single; Ki_d parameter double; lim parameter single; Ts parameter single; Kp_d parameter single; Ki_q parameter single; Kp_q parameter single
function [vd_out, vq_out, xid_next, xiq_next] = foc_vdq_pi_aw_min( ...
    id_ref, id_meas, iq_ref, iq_meas, ...
    C1, C2, xid, xiq, Ki_d, lim, Ts, ...
Kp_d, Ki_q, ...
Kp_q)
%#codegen
% MINIMO: PI(d,q) + C1/C2 + saturazione vettoriale + anti-windup back-calculation
% Stati integratori gestiti esternamente (Unit Delay / Discrete-Time Integrator)

% --- Anti-windup gain (regola pratica) ---
epsKp = single(1e-12);
Kaw_d = Ki_d / max(abs(Kp_d), epsKp);
Kaw_q = Ki_q / max(abs(Kp_q), epsKp);

% --- Errori ---
ed = id_ref - id_meas;
eq = iq_ref - iq_meas;

% --- PI + compensazioni (non saturato) ---
vd_unsat = (Kp_d * ed + xid) + C1;
vq_unsat = (Kp_q * eq + xiq) + C2;

% --- Saturazione vettoriale ---
Vmag  = sqrt(vd_unsat*vd_unsat + vq_unsat*vq_unsat);
Vsafe = max(Vmag, 1e-12);

k = lim / Vsafe;
if k > single(1)
    k = single(1);
elseif k < single(0)
    k = single(0);
end

vd_out = vd_unsat * k;
vq_out = vq_unsat * k;

% --- Anti-windup back-calculation ---
awd = vd_out - vd_unsat;
awq = vq_out - vq_unsat;

% --- Update integratori ---
xid_next = xid + Ts*(Ki_d*ed + Kaw_d*awd);
xiq_next = xiq + Ts*(Ki_q*eq + Kaw_q*awq);

end

== matlab function Simulation_full_Matlab/Controller/Control Loop/Measurament/MATLAB Function1 ==
  data: i1 input single; id output single; i2 input single; rho input single; iq output single
function [id, iq] = meas_fast(i1, i2, rho)
%#codegen
i1  = single(i1);
i2  = single(i2);
rho = single(rho);

inv_sqrt3 = single(0.5773502691896258); % 1/sqrt(3)

ialpha = i1;
ibeta  = inv_sqrt3 * (i1 + single(2)*i2);

c = cos(rho);
s = sin(rho);

id = ialpha*c + ibeta*s;
iq = ibeta*c - ialpha*s;
end

== matlab function Simulation_full_Matlab/Controller/Control Loop/Measurament/MATLAB Function3 ==
  data: is_d input; i_m_r output; Ts parameter; Tau_r parameter
function i_m_r = i_m_r_calculation(is_d, Ts, Tau_r)
%#codegen

persistent i_m_z
if isempty(i_m_z)
    i_m_z = single(0);
end

Tau_min = single(1e-6);
Tr = max(Tau_r, Tau_min);

i_m_z = i_m_z + (Ts/Tr) * (is_d - i_m_z);
i_m_r = i_m_z;
end

== matlab function Simulation_full_Matlab/Controller/Control Loop/Velocity_Flux_Loop/MATLAB Function ==
  settings: sampleTime=Ts*10
  data: i_s_d_rif input single; Up_limit_omega_1 output single; Is_adc parameter single; Down_limit_omega_1 output single
function [Up_limit_omega_1,Down_limit_omega_1]   = sqrt_max_diff(i_s_d_rif, Is_adc)

v = Is_adc*Is_adc - i_s_d_rif*i_s_d_rif;   % i_s_d_rif^2 - I_s_max^2
v = max(v, single(0));

Up_limit_omega_1 = sqrt(v);
Down_limit_omega_1=-Up_limit_omega_1;
end

== matlab function Simulation_full_Matlab/Controller/Control Loop/Current_Loop/MATLAB Function2 ==
  data: i_s_d input single; C_1 output single; i_s_q input single; i_mr_abs input single; w_r input single; C_2 output single; p parameter single; Tau_r parameter single; K_s parameter single; K_r parameter single
function [C_1, C_2] = fcn(i_s_d, i_s_q, i_mr_abs, w_r, p, Tau_r, K_s, K_r)
%#codegen

    critic_elem_1 = i_s_q / (Tau_r * i_mr_abs);
    critic_elem_2  = p * w_r + critic_elem_1;

    %--- Compensazioni (come schema AEAR)
    C_1 = (K_r/Tau_r) * (i_s_d - i_mr_abs) - K_s * i_s_q * critic_elem_2;
    C_2 = (K_s * i_s_d + K_r * i_mr_abs) * critic_elem_2;

end

== matlab function Simulation_full_Matlab/Controller/Control Loop/Refecence Funcion block/MATLAB Function ==
  data: wr input single; imr_ref output single; wr_n parameter single; imr_min parameter single
function imr_ref = imr_ref_from_wr(wr, wr_n, imr_min)
% wr     : velocità rotorica [rad/s]
% wr_n   : velocità base [rad/s] (deve essere >0)
% imr_ref_peak : corrente magnetizzante nominale (picco o dq coerente)
% imr_min: minimo ammesso

wr_abs  = abs(wr);
ref=single(35);
% Guardia su wr_n (evita wr_n=0/negativo/non inizializzato)
% if ~(isfinite(wr_n_abs) && wr_n_abs > 0)
%     imr_ref = imr_ref_peak;   % fallback: flusso nominale
%     return;
% end

if wr_abs <= wr_n
   imr_ref = ref;
else
   imr_ref = ref * (wr_n / wr_abs); % iperbolica
end

% % Guardia su avviamento / velocità ~0
% w_eps = 1e-3; % [rad/s] soglia (puoi alzare a 1e-2 se vuoi)
% if wr_abs < w_eps
%     imr_ref = single(25);
% else
%     if wr_abs <= wr_n_abs
%         imr_ref = single(25);
%     else
%         imr_ref = imr_ref_peak * (wr_n_abs / wr_abs); % iperbolica
%     end
% end

% % saturazione finale
imr_ref = max(imr_min, imr_ref);
end

== matlab function Simulation_full_Matlab/Controller/Control Loop/Velocity_Flux_Loop/MATLAB Function1 ==
  data: i_s_q_ref input single; Up_limit_PHI output single; Is_adc parameter
function Up_limit_PHI    = sqrt_max_diff(i_s_q_ref, Is_adc)

v = Is_adc*Is_adc - i_s_q_ref*i_s_q_ref;   % i_s_q_ref^2 - I_base_max^2
v = max(v, single(0));

Up_limit_PHI = sqrt(v);

end
